simulink model "pract3sl"  (R2024b)
settings: Solver=VariableStepAuto  StartTime=0.0  StopTime=10.0  RelTol=1e-3
InitFcn:
  | m1=290;
  | b1=1000;
  | m2=59;
  | k1=16182;
  | f=0;
  | k2=19000;
  | z1 =0.05;
  | z2 =0;
settings Model: Creator=sanch

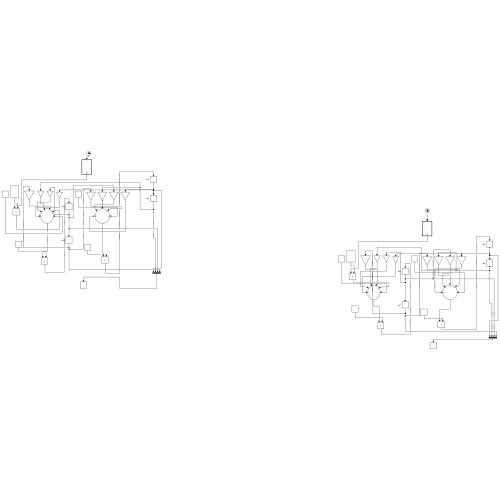
[thumbnail: Simulink's stored preview of the top-level diagram]
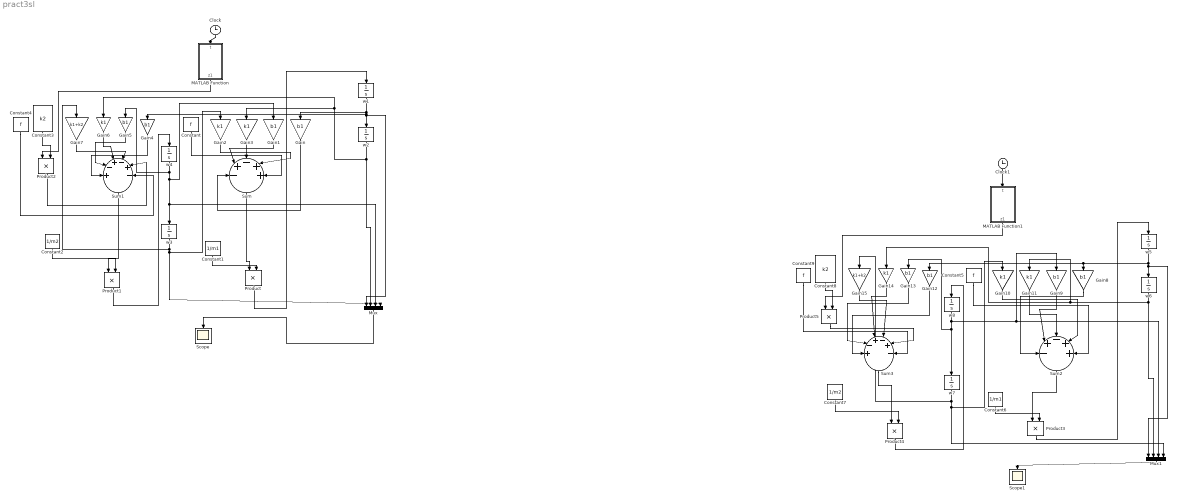
== system pract3sl ==
  Clock : Clock
  Clock1 : Clock
  Constant{,4..5,9} (4 alike) : Constant  Value=f
  Constant1 : Constant  Value=1/m1
  Constant2 : Constant  Value=1/m2
  Constant3 : Constant  Value=k2
  Constant6 : Constant  Value=1/m1
  Constant7 : Constant  Value=1/m2
  Constant8 : Constant  Value=k2
  Gain{,1,4..5,8..9,12..13} (8 alike) : Gain  Gain=b1
  Gain{2..3,6,10..11,14} (6 alike) : Gain  Gain=k1
  Gain15 : Gain  Gain=k1+k2
  Gain7 : Gain  Gain=k1+k2
  MATLAB Function : MATLAB Function  TreatAsAtomicUnit=on
  MATLAB Function1 : MATLAB Function  TreatAsAtomicUnit=on
  Mux : Mux
  Mux1 : Mux
  Product{,1..5} (6 alike) : Product
  Scope : Scope
  Scope1 : Scope
  Sum : Sum  Inputs=-+-++
  Sum1 : Sum  Inputs=+-+-+-
  Sum2 : Sum  Inputs=-+-++
  Sum3 : Sum  Inputs=+-+-+-
  w{1..8} (8 alike) : Integrator
  wires:
  Gain/1 -> Sum/1
  Gain1/1 -> Sum/2
  Gain3/1 -> Sum/3
  Gain2/1 -> Sum/4
  Mux/1 -> Scope/1
  Constant/1 -> Sum/5
  Sum/1 -> Product/1
  Constant1/1 -> Product/2
  Gain7/1 -> Sum1/4
  Gain6/1 -> Sum1/3
  Gain5/1 -> Sum1/2
  Gain4/1 -> Sum1/1
  Sum1/1 -> Product1/1
  Constant2/1 -> Product1/2
  Product1/1 -> w4/1
  w4/1 -> w3/1, Mux/3, Gain1/1, Gain5/1
  w3/1 -> Gain2/1, Mux/4, Gain7/1
  w1/1 -> w2/1, Mux/1, Gain4/1, Gain/1
  w2/1 -> Gain3/1, Gain6/1, Mux/2
  Product/1 -> w1/1
  Constant4/1 -> Sum1/6
  MATLAB Function/1(z1) -> Product2/1
  Constant3/1 -> Product2/2
  Product2/1 -> Sum1/5
  Clock/1 -> MATLAB Function/1(t)
  Constant7/1 -> Product4/2
  Gain12/1 -> Sum3/1
  Gain10/1 -> Sum2/4
  Gain14/1 -> Sum3/3
  Sum2/1 -> Product3/1
  Constant5/1 -> Sum2/5
  Gain9/1 -> Sum2/2
  w8/1 -> Gain13/1, w7/1, Mux1/3, Gain9/1
  Gain15/1 -> Sum3/4
  Gain8/1 -> Sum2/1
  Clock1/1 -> MATLAB Function1/1(t)
  Gain11/1 -> Sum2/3
  w7/1 -> Mux1/4, Gain10/1, Gain15/1
  Product4/1 -> w8/1
  Sum3/1 -> Product4/1
  Mux1/1 -> Scope1/1
  Constant6/1 -> Product3/2
  w5/1 -> w6/1, Mux1/1, Gain12/1, Gain8/1
  w6/1 -> Gain14/1, Gain11/1, Mux1/2
  Product3/1 -> w5/1
  Constant9/1 -> Sum3/6
  Gain13/1 -> Sum3/2
  MATLAB Function1/1(z1) -> Product5/1
  Constant8/1 -> Product5/2
  Product5/1 -> Sum3/5

== matlab function pract3sl/MATLAB Function ==
  data: t input; z1 output
function z1 = fcn(t)
z1= 0.05*sin(0.5*pi*t)
z2= 0.05*sin(20*pi*t)
%#codege

== matlab function pract3sl/MATLAB Function1 ==
  data: t input; z1 output
function z1 = fcn(t)
%z1= 0.05*sin(0.5*pi*t)
z1= 0.05*sin(20*pi*t)
%#codege
